simulink model "accelTestModel"  (Simulink 8.0)
settings: Solver=ode45  StartTime=0.0  StopTime=10.0  RelTol=1e-3
values from neighbouring files (symbols this model uses):
  beaver_init_p = 0    [beaver_4_14_2013.mat]    (also in monteCarloSim01.mat; simData_12_10_2013.mat; simData_12_9_2013.mat; simData_4_23_2013.mat)
  beaver_init_pitch = 0.13029612885    [beaver_4_14_2013.mat]    (also in monteCarloSim01.mat; simData_12_10_2013.mat; simData_12_9_2013.mat; simData_4_23_2013.mat)
  beaver_init_q = 0    [beaver_4_14_2013.mat]    (also in monteCarloSim01.mat; simData_12_10_2013.mat; simData_12_9_2013.mat; simData_4_23_2013.mat)
  beaver_init_r = 0    [beaver_4_14_2013.mat]    (also in monteCarloSim01.mat; simData_12_10_2013.mat; simData_12_9_2013.mat; simData_4_23_2013.mat)
  beaver_init_roll = 0    [beaver_4_14_2013.mat]    (also in monteCarloSim01.mat; simData_12_10_2013.mat; simData_12_9_2013.mat; simData_4_23_2013.mat)
libraries: aerolib6dof2 x1, aerolibnav x1
settings Model: Creator=atchase  LastModifiedBy=mufasa
settings DataIOCC: SignalLoggingSaveFormat=ModelDataLogs
settings DebuggingCC: FcnCallInpInsideContextMsg=EnableAllAsWarning
settings GRTTargetCC: CombineOutputUpdateFcns=off  GRTInterface=on

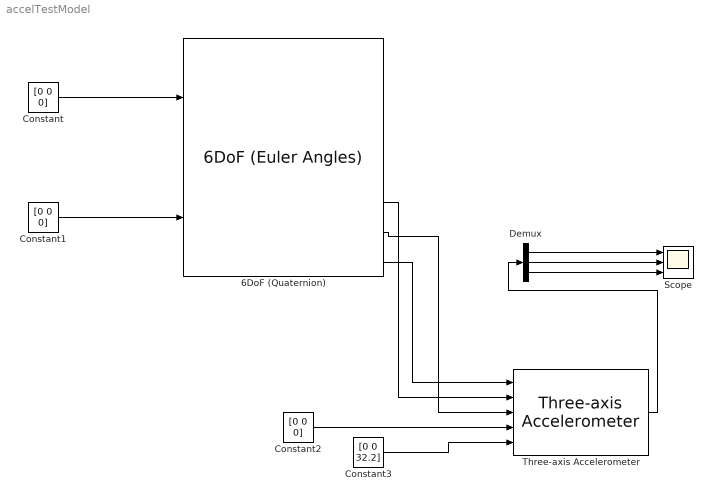
== system accelTestModel ==
  6DoF (Quaternion) : aerolib6dof2/6DoF (Euler Angles)  units=Metric (MKS)  mtype=Fixed  rep=Quaternion  xme_0=xme_0  Vm_0=[44.54 2.714 5.836]  eul_0=[beaver_init_roll, beaver_init_pitch, 113/180*pi]  pm_0=[beaver_init_p, beaver_init_q, beaver_init_r]  mass_0=beaver_mass  mass_e=0  mass_f=0  inertia="[5.787969e3  0 1.1764e2; 0 6.92893e3 0; -1.1764e2 0 1.1578329e4]"  inertia_e=eye(3)  inertia_f=eye(3)  k_quat=1.0
  Constant : Constant  Value=[0 0 0]
  Constant1 : Constant  Value=[0 0 0]
  Constant2 : Constant  Value=[0 0 0]
  Constant3 : Constant  Value=[0 0 32.2]
  Demux : Demux  Outputs=3
  Scope : Scope  NumInputPorts=3
      settings: TimeRange=10  YMin=-1~-1~-35  YMax=1~1~35
  Three-axis Accelerometer : aerolibnav/Three-axis Accelerometer  units=English  acc=[0 0 0]  gtype=on  dtype_a=on  w_a=190  z_a=0.707  a_sf_cc=[1 0 0; 0 1 0; 0 0 1]  a_bias=[0 0 0]  a_rand=on  a_seeds=[23093 23094 23095]  a_pow=[0.001 0.001 0.001]  a_sat="[-inf  -inf  -inf  inf inf inf]"  a_Ts=0
  wires:
  Constant/1 -> 6DoF (Quaternion)/1
  Constant1/1 -> 6DoF (Quaternion)/2
  6DoF (Quaternion)/8 -> Three-axis Accelerometer/1
  Demux/1 -> Scope/1
  Demux/2 -> Scope/2
  Demux/3 -> Scope/3
  6DoF (Quaternion)/6 -> Three-axis Accelerometer/2
  6DoF (Quaternion)/7 -> Three-axis Accelerometer/3
  Constant2/1 -> Three-axis Accelerometer/4
  Three-axis Accelerometer/1 -> Demux/1
  Constant3/1 -> Three-axis Accelerometer/5
